simulink model "MicoArchitecture"  (R2017a)
settings: Solver=VariableStepAuto  StartTime=0.0  StopTime=10.0  RelTol=1e-3
values from neighbouring files (symbols this model uses):
  a = 127*rand(384,1)    [Infup for Xilinx Hardware.m]    (also in Input_for_Xilinx_Hardware.m)
undefined symbols (not defined in the file or in its folder): b, c
libraries: simulink_extras x7, simulink x2, hdlsllib x2
settings Model: Creator=HAZOOR  LastModifiedBy=HAZOOR

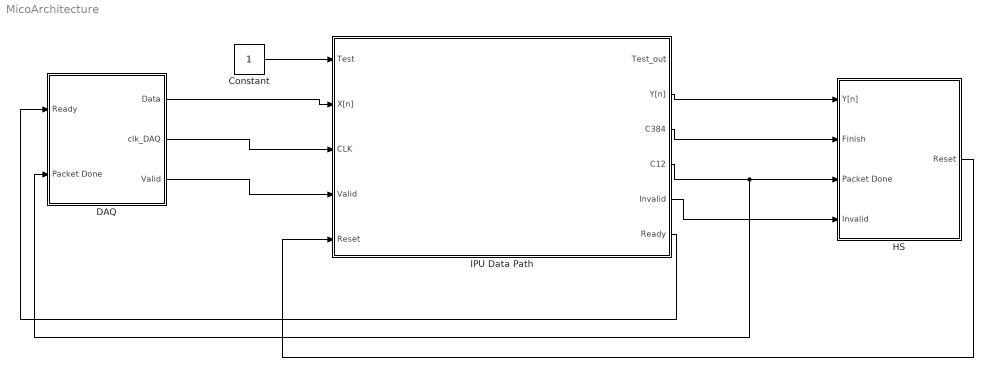
== system MicoArchitecture ==
  Constant : Constant  SampleTime=10
  DAQ : Subsystem
  HS : Subsystem
  IPU Data Path : Subsystem
  wires:
  IPU Data Path/4(C12) -> HS/3(Packet Done), DAQ/2(Packet Done)
  DAQ/1(Data) -> IPU Data Path/2(X[n])
  Constant/1 -> IPU Data Path/1(Test)
  DAQ/2(clk_DAQ) -> IPU Data Path/3(CLK)
  IPU Data Path/2(Y[n]) -> HS/1(Y[n])
  DAQ/3(Valid) -> IPU Data Path/4(Valid)
  IPU Data Path/5(Invalid) -> HS/4(Invalid)
  IPU Data Path/3(C384) -> HS/2(Finish)
  HS/1(Reset) -> IPU Data Path/5(Reset)
  IPU Data Path/6(Ready) -> DAQ/1(Ready)

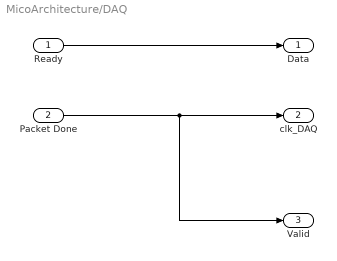
== system MicoArchitecture/DAQ ==
  Ready : Inport
  Packet Done : Inport  Port=2
  Data : Outport
  clk_DAQ : Outport  Port=2
  Valid : Outport  Port=3
  wires:
  Ready/1 -> Data/1
  Packet Done/1 -> Valid/1, clk_DAQ/1

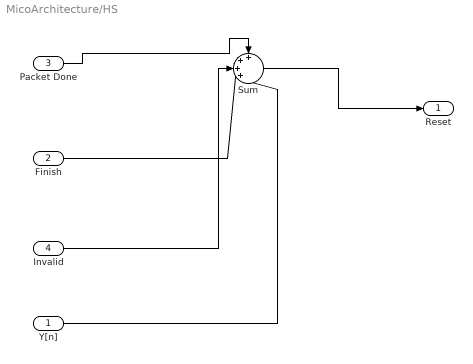
== system MicoArchitecture/HS ==
  Y[n] : Inport
  Finish : Inport  Port=2
  Packet Done : Inport  Port=3
  Invalid : Inport  Port=4
  Sum : Sum  Inputs=++++|
  Reset : Outport
  wires:
  Packet Done/1 -> Sum/1
  Finish/1 -> Sum/2
  Sum/1 -> Reset/1
  Invalid/1 -> Sum/3
  Y[n]/1 -> Sum/4

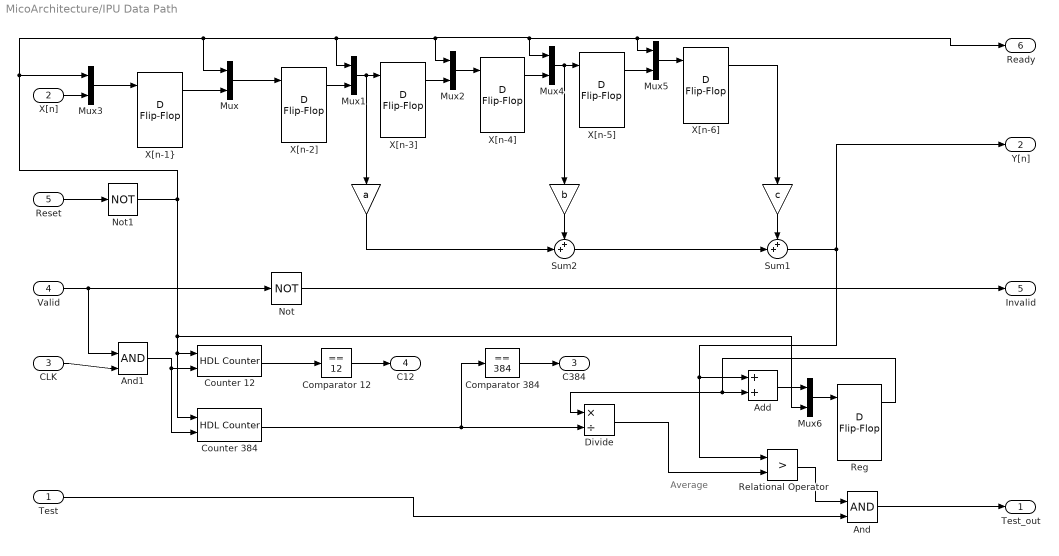
== system MicoArchitecture/IPU Data Path ==
  note: Average
  Test : Inport
  X[n] : Inport  Port=2
  CLK : Inport  Port=3
  Valid : Inport  Port=4
  Reset : Inport  Port=5
  " " : Gain  Gain=a
  "  " : Gain  Gain=b
  "   " : Gain  Gain=c
  Add : Sum
  And : Logic  IconShape=distinctive  AllPortsSameDT=off  OutDataTypeStr=boolean
  And1 : Logic  IconShape=distinctive  AllPortsSameDT=off  OutDataTypeStr=boolean
  Comparator 12 : simulink/Logic and Bit Operations/Compare To Constant  relop===  const=12  OutDataTypeStr=boolean
  Comparator 384 : simulink/Logic and Bit Operations/Compare To Constant  relop===  const=384  OutDataTypeStr=boolean
  Counter 12 : hdlsllib/HDL Operations/HDL Counter  CountType=Count limited  CountInit=0  CountStep=1  CountMax=11  CountFromType=Initial value  CountFrom=0  CountResetPort=on  CountLoadPort=off  CountEnbPort=on  CountDirPort=off  CountDataType=Unsigned  CountWordLen=8  CountFracLen=0  CountSampTime=1
      settings: SourceProductName=HDL Coder  SourceProductBaseCode=HD
  Counter 384 : hdlsllib/HDL Operations/HDL Counter  CountType=Count limited  CountInit=0  CountStep=1  CountMax=384  CountFromType=Initial value  CountFrom=0  CountResetPort=on  CountLoadPort=off  CountEnbPort=on  CountDirPort=off  CountDataType=Unsigned  CountWordLen=32  CountFracLen=0  CountSampTime=1
      settings: SourceProductName=HDL Coder  SourceProductBaseCode=HD
  Divide : Product  Inputs=*/
  Mux{,1..6} (7 alike) : Mux  Inputs=2
  Not : Logic  Operator=NOT  IconShape=distinctive  AllPortsSameDT=off  OutDataTypeStr=boolean
  Not1 : Logic  Operator=NOT  IconShape=distinctive  AllPortsSameDT=off  OutDataTypeStr=boolean
  "Reg " : simulink_extras/Flip Flops/D Flip-Flop
      settings: SourceProductName=Simulink
  Relational Operator : RelationalOperator  Operator=>  OutDataTypeStr=boolean  RndMeth=Simplest
  Sum1 : Sum  Inputs=++|
  Sum2 : Sum  Inputs=++|
  "X[n-1}" : simulink_extras/Flip Flops/D Flip-Flop
      settings: SourceProductName=Simulink
  X[n-2] : simulink_extras/Flip Flops/D Flip-Flop
      settings: SourceProductName=Simulink
  X[n-3] : simulink_extras/Flip Flops/D Flip-Flop
      settings: SourceProductName=Simulink
  X[n-4] : simulink_extras/Flip Flops/D Flip-Flop
      settings: SourceProductName=Simulink
  X[n-5] : simulink_extras/Flip Flops/D Flip-Flop
      settings: SourceProductName=Simulink
  X[n-6] : simulink_extras/Flip Flops/D Flip-Flop
      settings: SourceProductName=Simulink
  Test_out : Outport
  Y[n] : Outport  Port=2
  C384 : Outport  Port=3
  C12 : Outport  Port=4
  Invalid : Outport  Port=5
  Ready : Outport  Port=6
  wires:
  Sum1/1 -> Relational Operator/1, Add/1, Y[n]/1
  Counter 12/1 -> Comparator 12/1
  Test/1 -> And/2
  And/1 -> Test_out/1
  Counter 384/1 -> Comparator 384/1, Divide/2
  Comparator 12/1 -> C12/1
  Comparator 384/1 -> C384/1
  Divide/1 -> Relational Operator/2
  "  "/1 -> Sum2/1
  " "/1 -> Sum2/2
  "   "/1 -> Sum1/1
  Sum2/1 -> Sum1/2
  "Reg "/1 -> Divide/1, Add/2
  X[n-6]/1 -> "   "/1
  Relational Operator/1 -> And/1
  CLK/1 -> And1/2
  And1/1 -> Counter 384/2, Counter 12/2
  Valid/1 -> Not/1, And1/1
  Not/1 -> Invalid/1
  Reset/1 -> Not1/1
  Not1/1 -> Mux6/2, Counter 384/1, Counter 12/1, Mux3/1, Mux/1, Mux1/1, Mux2/1, Ready/1, Mux5/1, Mux4/1
  Mux/1 -> X[n-2]/1
  "X[n-1}"/1 -> Mux/2
  Mux1/1 -> " "/1, X[n-3]/1
  X[n-2]/1 -> Mux1/2
  X[n-3]/1 -> Mux2/2
  Mux2/1 -> X[n-4]/1
  X[n]/1 -> Mux3/2
  Mux3/1 -> "X[n-1}"/1
  X[n-4]/1 -> Mux4/2
  Mux4/1 -> "  "/1, X[n-5]/1
  X[n-5]/1 -> Mux5/2
  Mux5/1 -> X[n-6]/1
  Mux6/1 -> "Reg "/1
  Add/1 -> Mux6/1
